simulink model "PSA_final"  (R2020a)
settings: Solver=ode45  StartTime=0.0  StopTime=1  RelTol=1e-3  EnableMultiTasking=on
settings Model: Creator=Zero  LastModifiedBy=hp
settings DataIOCC: LimitDataPoints=on  SaveFormat=Array  ReturnWorkspaceOutputs=off
settings OptimizationCC: LifeSpan=inf
settings DebuggingCC: SolverPrmCheckMsg=warning  SFUnexpectedBacktrackingDiag=warning  SFNoUnconditionalDefaultTransitionDiag=warning  SFExecutionAtInitializationDiag=none  ArithmeticOperatorsInVariantConditions=warning
settings HardwareCC: ProdBitPerPointer=32  ProdBitPerSizeT=32  ProdBitPerPtrDiffT=32  ProdLargestAtomicFloat=None  ProdIntDivRoundTo=Undefined  ProdEndianess=Unspecified  ProdWordSize=32  ProdHWDeviceType=32-bit Generic
settings ModelReferenceCC: PropagateSignalLabelsOutOfModel=off
settings SFSimCC: SimUseLocalCustomCode=off  CustomCodeUndefinedFunction=UseInterfaceOnly
settings RTWCC: RTWUseLocalCustomCode=off
settings CodeAppCC: StateflowObjectComments=on
settings GRTTargetCC: TargetLangStandard=C89/C90 (ANSI)
settings ConfigComp: CovMetricSettings=dw  CovHtmlReporting=on  CovSaveCumulativeToWorkspaceVar=on  CovSaveSingleToWorkspaceVar=on  CovExternalEMLEnable=off  CovSFcnEnable=off

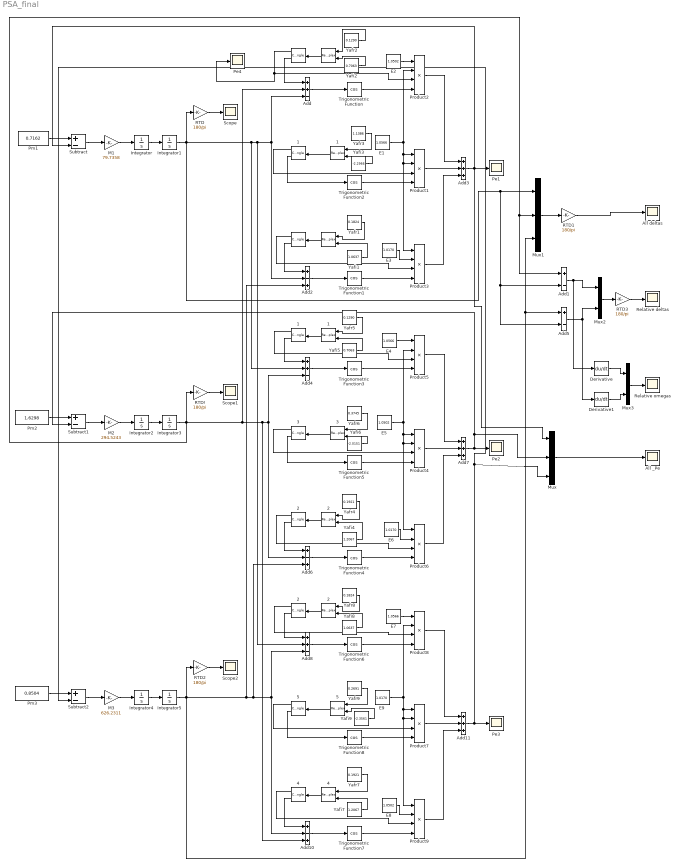
== system PSA_final ==
   {,,1,1..2,2..5} (9 alike) : ComplexToMagnitudeAngle
   {,,1,1..2,2..5} (9 alike) : RealImagToComplex
  Add : Sum  Inputs=++-
  Add1 : Sum  Inputs=+-
  Add10 : Sum  Inputs=+-+
  Add11 : Sum  Inputs=+++
  Add2 : Sum  Inputs=+-+
  Add3 : Sum  Inputs=+++
  Add4 : Sum  Inputs=++-
  Add5 : Sum  Inputs=+-
  Add6 : Sum  Inputs=+-+
  Add7 : Sum  Inputs=+++
  Add8 : Sum  Inputs=++-
  All _Pe : Scope
  All deltas : Scope
  Derivative : Derivative
  Derivative1 : Derivative
  E1 : Constant  Value=1.0566
  E2 : Constant  Value=1.0502
  E3 : Constant  Value=1.0170
  E4 : Constant  Value=1.0566
  E5 : Constant  Value=1.0502
  E6 : Constant  Value=1.0170
  E7 : Constant  Value=1.0566
  E8 : Constant  Value=1.0502
  E9 : Constant  Value=1.0170
  Integrator{,1..5} (6 alike) : Integrator
  M1 : Gain  Gain=79.7358
  M2 : Gain  Gain=294.5243
  M3 : Gain  Gain=626.2311
  Mux : Mux  Inputs=3
  Mux1 : Mux  Inputs=3
  Mux2 : Mux  Inputs=2
  Mux3 : Mux  Inputs=2
  Pe{1..4} (4 alike) : Scope
  Pm1 : Constant  Value=0.7162
  Pm2 : Constant  Value=1.6298
  Pm3 : Constant  Value=0.8504
  Product{1..9} (9 alike) : Product  Inputs=4
  RTD{,1..3} (4 alike) : Gain  Gain=180/pi
  RTD! : Gain  Gain=180/pi
  Relative deltas : Scope
  "Relative omegas " : Scope
  Scope : Scope
  Scope1 : Scope
  Scope2 : Scope
  Subtract : Sum  Inputs=+-
  Subtract1 : Sum  Inputs=+-
  Subtract2 : Sum  Inputs=+-
  Trigonometric Function{,1..8} (9 alike) : Trigonometry  Operator=cos
  Yafi1 : Constant  Value=1.0637
  Yafi2 : Constant  Value=0.7063
  Yafi3 : Constant  Value=-2.2966
  Yafi4 : Constant  Value=1.2067
  Yafi5 : Constant  Value=0.7063
  Yafi6 : Constant  Value=-2.0151
  Yafi7 : Constant  Value=1.2067
  Yafi8 : Constant  Value=1.0637
  Yafi9 : Constant  Value=-2.3561
  Yafr1 : Constant  Value=0.1824
  Yafr2 : Constant  Value=0.1290
  Yafr3 : Constant  Value=1.1386
  Yafr4 : Constant  Value=0.1921
  Yafr5 : Constant  Value=0.1290
  Yafr6 : Constant  Value=0.3745
  Yafr7 : Constant  Value=0.1921
  Yafr8 : Constant  Value=0.1824
  Yafr9 : Constant  Value=0.2691
  wires:
  " "/2 -> Add2/1
  " "/1 -> " "/1
  Add2/1 -> Trigonometric Function1/1
  " "/1 -> Product3/3
  Pm1/1 -> Subtract/1
  Subtract/1 -> M1/1
  M1/1 -> Integrator/1
  Integrator/1 -> Integrator1/1
  RTD/1 -> Scope/1
  E3/1 -> Product3/2
  " "/1 -> " "/1
  " "/2 -> Add/1
  Add/1 -> Trigonometric Function/1
  Trigonometric Function1/1 -> Product3/4
  Trigonometric Function/1 -> Product2/4
  " "/1 -> Pe4/1, Product2/3
  " 1"/1 -> " 1"/1
  " 1"/2 -> Trigonometric Function2/1
  Trigonometric Function2/1 -> Product1/4
  " 1"/1 -> Product1/3
  E1/1 -> Product3/1, Product1/2, Product1/1, Product2/2
  Product1/1 -> Add3/2
  Product2/1 -> Add3/1
  Product3/1 -> Add3/3
  Add3/1 -> Mux/1, Pe1/1, Subtract/2
  " 2"/2 -> Add6/1
  " 2"/1 -> " 2"/1
  Add6/1 -> Trigonometric Function4/1
  " 2"/1 -> Product6/3
  Pm2/1 -> Subtract1/1
  Subtract1/1 -> M2/1
  M2/1 -> Integrator2/1
  Integrator2/1 -> Integrator3/1
  RTD!/1 -> Scope1/1
  E6/1 -> Product6/2
  " 1"/1 -> " 1"/1
  " 1"/2 -> Add4/1
  Add4/1 -> Trigonometric Function3/1
  Trigonometric Function4/1 -> Product6/4
  Trigonometric Function3/1 -> Product5/4
  " 1"/1 -> Product5/3
  " 3"/1 -> " 3"/1
  " 3"/2 -> Trigonometric Function5/1
  Trigonometric Function5/1 -> Product4/4
  " 3"/1 -> Product4/3
  E4/1 -> Product5/1
  E5/1 -> Product6/1, Product4/2, Product4/1, Product5/2
  Product4/1 -> Add7/2
  Product5/1 -> Add7/1
  Product6/1 -> Add7/3
  Add7/1 -> Mux/2, Subtract1/2, Pe2/1
  " 4"/2 -> Add10/1
  " 4"/1 -> " 4"/1
  Add10/1 -> Trigonometric Function7/1
  " 4"/1 -> Product9/3
  Pm3/1 -> Subtract2/1
  Subtract2/1 -> M3/1
  M3/1 -> Integrator4/1
  Integrator4/1 -> Integrator5/1
  RTD2/1 -> Scope2/1
  E8/1 -> Product9/2
  " 2"/1 -> " 2"/1
  " 2"/2 -> Add8/1
  Add8/1 -> Trigonometric Function6/1
  Trigonometric Function7/1 -> Product9/4
  Trigonometric Function6/1 -> Product8/4
  " 2"/1 -> Product8/3
  " 5"/1 -> " 5"/1
  " 5"/2 -> Trigonometric Function8/1
  Trigonometric Function8/1 -> Product7/4
  " 5"/1 -> Product7/3
  E7/1 -> Product8/1
  E9/1 -> Product9/1, Product7/2, Product7/1, Product8/2
  Product7/1 -> Add11/2
  Product8/1 -> Add11/1
  Product9/1 -> Add11/3
  Add11/1 -> Pe3/1, Mux/3, Subtract2/2
  Integrator5/1 -> Add5/1, Mux1/3, RTD2/1, Add2/3, Add6/3, Add8/3, Add10/2
  Integrator3/1 -> Add1/1, Mux1/2, RTD!/1, Add/2, Add10/3, Add6/2, Add4/3
  Yafi2/1 -> " "/2
  Yafr2/1 -> " "/1
  Yafi3/1 -> " 1"/2
  Yafr3/1 -> " 1"/1
  Yafi1/1 -> " "/2
  Yafr1/1 -> " "/1
  E2/1 -> Product2/1
  Yafi6/1 -> " 3"/2
  Yafr6/1 -> " 3"/1
  Yafi5/1 -> " 1"/2
  Yafr5/1 -> " 1"/1
  Yafi4/1 -> " 2"/2
  Yafr4/1 -> " 2"/1
  Yafi9/1 -> " 5"/2
  Yafr9/1 -> " 5"/1
  Yafi8/1 -> " 2"/2
  Yafr8/1 -> " 2"/1
  Yafi7/1 -> " 4"/2
  Yafr7/1 -> " 4"/1
  Mux/1 -> All _Pe/1
  Mux1/1 -> RTD1/1
  RTD1/1 -> All deltas/1
  Add1/1 -> Derivative/1, Mux2/1
  Add5/1 -> Mux2/2, Derivative1/1
  Integrator1/1 -> Add5/2, Add1/2, Mux1/1, RTD/1, Add4/2, Add8/2, Add/3, Add2/2
  RTD3/1 -> Relative deltas/1
  Mux2/1 -> RTD3/1
  Derivative/1 -> Mux3/1
  Derivative1/1 -> Mux3/2
  Mux3/1 -> "Relative omegas "/1
